simulink model "RI_RL_PI_AW"  (R2013b)
settings: Solver=ode45  StartTime=0.0  StopTime=20e-3  MaxStep=tau/100  RelTol=1e-3
InitFcn:
  | % Modellparaméterek
  | R = 250e-3;
  | L = 10e-3;
  | Psi_0 = 0.5e-3;
  | 
  | i_0 = 0;
  | theta_0 = 0;
  | 
  | % Rendszerparaméterek
  | K = 1/R;
  | tau = L/R;
  | 
  | % PI-hangolás
  | tau_CL = tau/25;
  | xi_CL = 1;
  | 
  | K_PI = (2*xi_CL*tau - tau_CL)/(K*tau_CL);
  | T_I = (2*xi_CL*tau - tau_CL)*tau_CL/tau;
libraries: RI_MK x2
settings Model: Creator=Szalay  LastModifiedBy=Szalay

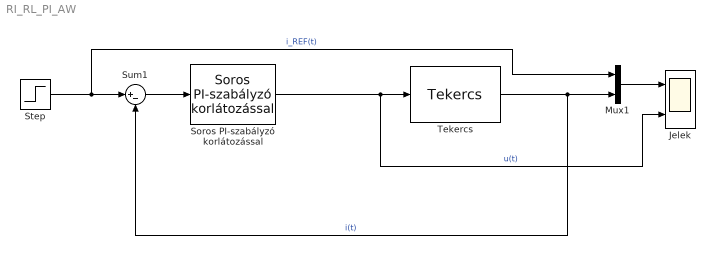
== system RI_RL_PI_AW ==
  Jelek : Scope  NumInputPorts=2
      settings: ShowLegends=on  TimeRange=0.02  YMin=0~-1  YMax=0.7000000000000001~8
  Mux1 : Mux  Inputs=2
  Soros PI-szabályzó korlátozással : RI_MK/Soros PI-szabályzó korlátozással  K_PI=K_PI  T_I=T_I  L_U=5  L_L=-5  T_T=T_I
  Step : Step  Time=5e-3  After=0.6  SampleTime=0
  Sum1 : Sum  Inputs=|+-
  Tekercs : RI_MK/Tekercs  R=R  L=L  i_0=i_0
  wires:
  Mux1/1 -> Jelek/1
  Soros PI-szabályzó korlátozással/1 -> Jelek/2, Tekercs/1  "u(t)"
  Step/1 -> Mux1/1, Sum1/1  "i_REF(t)"
  Tekercs/1 -> Sum1/2, Mux1/2  "i(t)"
  Sum1/1 -> Soros PI-szabályzó korlátozással/1
